simulink model "protocol"  (R2025b)
settings: Solver=FixedStepDiscrete  StartTime=0.0  StopTime=20  RelTol=1e-3
settings Model: NumberOfSteps=5  Creator=Dell  LastModifiedBy=Dell

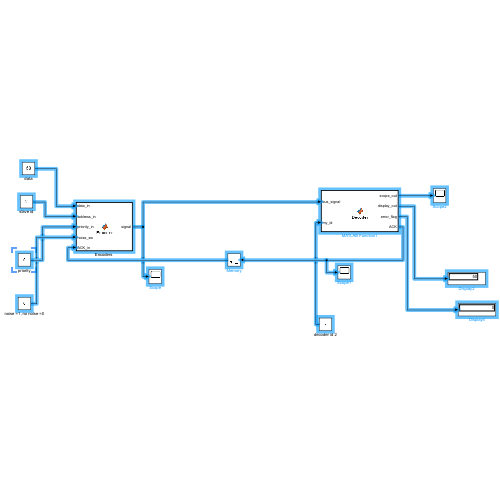
[thumbnail: Simulink's stored preview of the top-level diagram]
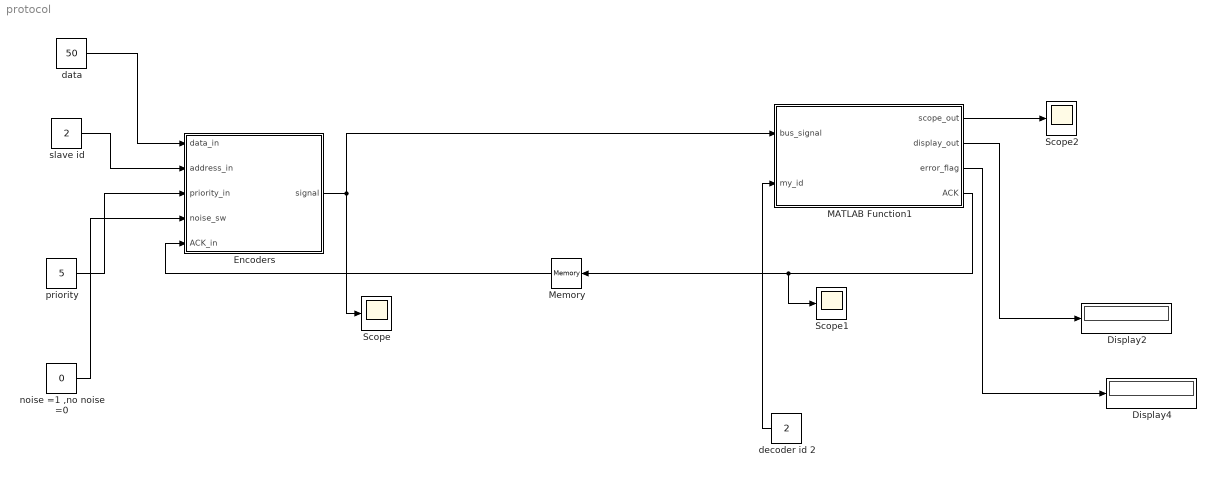
== system protocol ==
  Display2 : Display
  Display4 : Display
      settings: Format=decimal (Stored Integer)
  "Encoders " : MATLAB Function  TreatAsAtomicUnit=on
  MATLAB Function1 : MATLAB Function  TreatAsAtomicUnit=on
  Memory : Memory
  Scope : Scope
      settings: SampleTime=0.05  TimeSpan=4.1  ActiveDisplayYMinimum=-0.62499999999999989  ActiveDisplayYMaximum=5.625  DataLoggingVariableName=ScopeData2  DataLoggingSaveFormat=Array
  Scope1 : Scope
      settings: ActiveDisplayYMinimum=1.1153884061838302  ActiveDisplayYMaximum=1.67249261744699  DataLoggingSaveFormat=Array
  Scope2 : Scope
      settings: SampleTime=0.05  TimeSpan=4.1  ActiveDisplayYMinimum=-0.62499999999999989  ActiveDisplayYMaximum=5.625  DataLoggingSaveFormat=Array
  data : Constant  Value=50
  decoder id 2 : Constant  Value=2
  noise =1 ,no noise =0 : Constant  Value=0
  priority : Constant  Value=5
  slave id : Constant  Value=2
  wires:
  MATLAB Function1/2(display_out) -> Display2/1
  decoder id 2/1 -> MATLAB Function1/2(my_id)
  MATLAB Function1/1(scope_out) -> Scope2/1
  data/1 -> "Encoders "/1(data_in)
  slave id/1 -> "Encoders "/2(address_in)
  priority/1 -> "Encoders "/3(priority_in)
  MATLAB Function1/3(error_flag) -> Display4/1
  "Encoders "/1(signal) -> Scope/1, MATLAB Function1/1(bus_signal)
  Memory/1 -> "Encoders "/5(ACK_in)
  MATLAB Function1/4(ACK) -> Scope1/1, Memory/1
  noise =1 ,no noise =0/1 -> "Encoders "/4(noise_sw)

== matlab function protocol/Encoders  ==
  settings: updateMethod=DISCRETE  sampleTime=0.05
  data: data_in input; signal output; address_in input; priority_in input; noise_sw input; ACK_in input
function signal = Encoder(data_in, address_in, priority_in, noise_sw, ACK_in)
    persistent full_frame frame_index ack_buffer noise_done prev_noise_sw;

    if isempty(frame_index)
        frame_index   = int32(1);
        ack_buffer    = zeros(1,16);
        noise_done    = int32(0);
        prev_noise_sw = double(-1);
        full_frame    = zeros(1,80);
    end

    fi = double(frame_index);

    if noise_sw ~= prev_noise_sw
        noise_done    = int32(0);
        ack_buffer    = zeros(1,16);
        prev_noise_sw = double(noise_sw);
    end

    if fi >= 39 && fi <= 54
        ack_pos = fi - 38;
        if ack_pos >= 1 && ack_pos <= 16
            if ACK_in == 5
                ack_buffer(ack_pos) = double(1);
            else
                ack_buffer(ack_pos) = double(0);
            end
        end
    end

    if frame_index == int32(1)
        if noise_sw == 0
            full_frame = BuildFrame(data_in, address_in, priority_in, 0);

        elseif noise_sw == 1
            if noise_done == int32(0)
                full_frame = BuildFrame(data_in, address_in, priority_in, 1);
            else
                full_frame = BuildFrame(data_in, address_in, priority_in, 0);
            end

        elseif noise_sw == 2
            full_frame = BuildFrame(data_in, address_in, priority_in, 1);
        end
    end

    if frame_index == int32(80)
        if noise_sw == 1
            high_count = sum(ack_buffer);

            if high_count == 16
                % ALL HIGH: OK, data was clean
                noise_done = int32(1);

            elseif high_count == 0
                % ALL LOW: ERROR, noise detected, switch to clean
                noise_done = int32(1);

            else
                % MIXED: corruption, keep retrying
                noise_done = int32(0);
            end
        end

        ack_buffer  = zeros(1,16);
        frame_index = int32(1);
    end

    signal = full_frame(double(frame_index));

    if frame_index < int32(80)
        frame_index = frame_index + int32(1);
    end

end

function full_frame = BuildFrame(data_in, address_in, priority_in, use_noise)
    data_bits = double(bitget(uint8(data_in),     8:-1:1));
    addr_bits = double(bitget(uint8(address_in),  8:-1:1));
    prio_bits = double(bitget(uint8(priority_in), 8:-1:1));

    payload = reshape([data_bits; data_bits], 1, []);

    if use_noise == 1
        noise_idx = randi([1,16], 1, 2);
        for i = noise_idx
            payload(i) = double(~logical(payload(i)));
        end
    end

    header         = [1, 0];
    prio_block     = [prio_bits, 0];
    addr_block     = [addr_bits, 0];
    data_start_gap = zeros(1,20);
    data_block     = payload;
    data_end_gap   = zeros(1,20);
    tail           = [0, 1, 0, 0];

    logic_seq  = [header, prio_block, addr_block, data_start_gap, data_block, data_end_gap, tail];
    full_frame = logic_seq * 5;
end

== matlab function protocol/MATLAB Function1 ==
  settings: updateMethod=DISCRETE  sampleTime=0.05
  data: scope_out output; bus_signal input; my_id input; display_out output; error_flag output; ACK output
function [scope_out, display_out, error_flag, ACK] = Decoder(bus_signal, my_id)
    persistent state bit_count addr_buffer result mat_a mat_b err_flag ack_frame ack_index in_gap ack_sending;

    if isempty(state)
        state       = int32(0);
        bit_count   = int32(0);
        addr_buffer = zeros(1,8);
        result      = double(0);
        mat_a       = zeros(1,8);
        mat_b       = zeros(1,8);
        err_flag    = double(0);
        ack_frame   = zeros(1,20);
        ack_index   = int32(0);
        in_gap      = int32(0);
        ack_sending = int32(0);
    end

    is_high   = double(bus_signal == 5);
    scope_out = double(0);
    ACK       = double(0);

    switch state

        case 0
            if ack_sending == int32(1)
                if ack_index >= int32(1) && ack_index <= int32(20)
                    ACK       = ack_frame(double(ack_index));
                    ack_index = ack_index + int32(1);
                else
                    ack_sending = int32(0);
                    ack_index   = int32(0);
                end
            else
                if is_high
                    state     = int32(1);
                    bit_count = int32(0);
                end
            end

        case 1
            bit_count = bit_count + int32(1);
            if bit_count >= int32(10)
                state       = int32(2);
                bit_count   = int32(0);
                addr_buffer = zeros(1,8);
            end

        case 2
            bit_count = bit_count + int32(1);
            idx = double(bit_count);
            if idx <= 8
                addr_buffer(idx) = is_high;
            end
            if bit_count == int32(8)
                received_id = sum(addr_buffer .* 2.^(7:-1:0));
                if received_id == double(my_id)
                    state     = int32(3);
                    bit_count = int32(0);
                    mat_a     = zeros(1,8);
                    mat_b     = zeros(1,8);
                else
                    state = int32(0);
                end
            end

        case 3
            bit_count = bit_count + int32(1);
            scope_out = double(bus_signal);

            data_pos = double(bit_count) - 21.0;
            if data_pos >= 1.0 && data_pos <= 16.0
                pair_index = ceil(data_pos / 2.0);
                if mod(data_pos, 2.0) == 1.0
                    mat_a(pair_index) = is_high;
                else
                    mat_b(pair_index) = is_high;
                end
            end

            if bit_count == int32(38)
                if all(mat_a == mat_b)
                    % OK: all 16 bits high = 11111111 11111111
                    result   = double(sum(mat_a .* 2.^(7:-1:0)));
                    err_flag = double(0);
                    ack_bits = [1,1,1,1,1,1,1,1]; % ALL HIGH = OK
                else
                    % ERROR: all 16 bits low = 00000000 00000000
                    result   = double(0);
                    err_flag = double(1);
                    ack_bits = [0,0,0,0,0,0,0,0]; % ALL LOW = ERROR
                end
                ack_doubled = reshape([ack_bits; ack_bits], 1, []) * 5;
                ack_frame   = [ack_doubled, zeros(1,4)];
                ack_index   = int32(1);
                in_gap      = int32(1);
            end

            if in_gap == int32(1)
                if ack_index >= int32(1) && ack_index <= int32(20)
                    ACK       = ack_frame(double(ack_index));
                    ack_index = ack_index + int32(1);
                else
                    in_gap = int32(0);
                end
            end

            if bit_count >= int32(61)
                if ack_index >= int32(1) && ack_index <= int32(20)
                    ack_sending = int32(1);
                else
                    ack_sending = int32(0);
                    ack_index   = int32(0);
                end
                in_gap = int32(0);
                state  = int32(0);
            end

    end

    display_out = result;
    error_flag  = err_flag;

end
